simulink model "sim10"  (R2022b)
settings: Solver=VariableStepAuto  StartTime=0.0  StopTime=czas_symulacji  RelTol=1e-3
values from neighbouring files (symbols this model uses):
  Cvp = cp*rop*Vp    (= 36000)    [Lab5.m]    (also in Lab5_wspolne_wykresy.m)
  Cvw = cp*rop*Vw    (= 67200)    [Lab5.m]    (also in Lab5_wspolne_wykresy.m)
  dqg = 0.1*qgN    (= 1000)    [Lab5.m]    (also in Lab5_wspolne_wykresy.m)
  dTzew = 1    [Lab5.m]    (also in Lab5_wspolne_wykresy.m)
  kcp = (a*qgN*(TwewN-TpN))/((TpN-TzewN)*((TwewN-TzewN)+a*(TwewN-TpN)))    (= 23.2558139535)    [Lab5.m]    (also in Lab5_wspolne_wykresy.m)
  kcw = qgN/((TwewN-TzewN)+a*(TwewN-TpN))    (= 232.558139535)    [Lab5.m]    (also in Lab5_wspolne_wykresy.m)
  kcwp = a*kcw    (= 69.7674418605)    [Lab5.m]    (also in Lab5_wspolne_wykresy.m)
  L11 = M2    [Lab5.m]    (also in Lab5_wspolne_wykresy.m)
  L12 = [kcw*Cvp kcp*kcwp+kcw*kcwp+kcw*kcp]    [Lab5.m]    (also in Lab5_wspolne_wykresy.m)
  L21 = kcwp    (= 69.7674418605)    [Lab5.m]    (also in Lab5_wspolne_wykresy.m)
  L22 = [kcp*Cvw kcwp*kcw+kcw*kcp+kcwp*kcp]    [Lab5.m]    (also in Lab5_wspolne_wykresy.m)
  M = [Cvw*Cvp Cvw*kcwp+Cvw*kcp+Cvp*kcw+Cvp*kcwp kcw*kcwp+kcw*kcp+kcwp*kcp]    [Lab5.m]    (also in Lab5_wspolne_wykresy.m)
  qg0 = X(i)    [Lab5.m]    (also in Lab5_wspolne_wykresy.m)
  t0 = 1000    [Lab5.m]    (also in Lab5_wspolne_wykresy.m)
  Tp0 = ((kcp*Tzew0)*(kcw+kcwp)+kcwp*(qg0+kcw*Tzew0))/(kcwp*kcw+kcp*kcw+kcp*kcwp)    [Lab5.m]    (also in Lab5_wspolne_wykresy.m)
  Twew0 = (qg0+kcw*Tzew0+kcwp*Tp0)/(kcw+kcwp)    [Lab5.m]    (also in Lab5_wspolne_wykresy.m)
  Tzew0 = Y(i)    [Lab5.m]    (also in Lab5_wspolne_wykresy.m)
settings Model: Creator=franc  LastModifiedBy=Dawkin
settings DataIOCC: ReturnWorkspaceOutputs=off

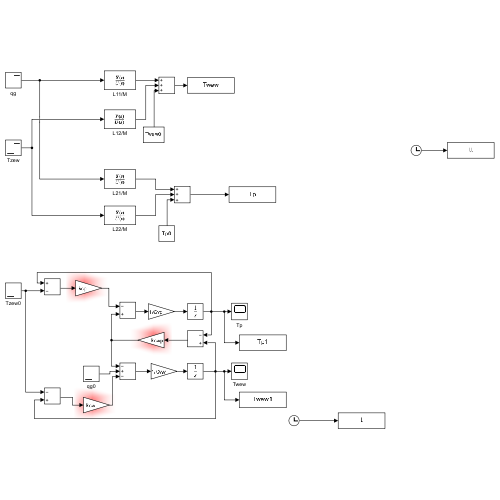
[thumbnail: Simulink's stored preview of the top-level diagram]
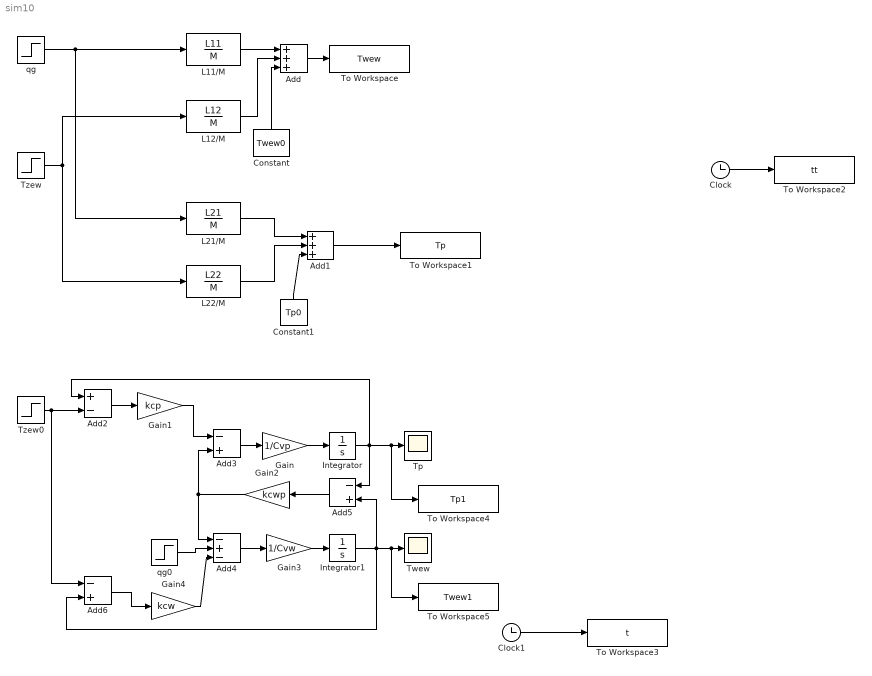
== system sim10 ==
  Add : Sum  Inputs=+++
  Add1 : Sum  Inputs=+++
  Add2 : Sum  Inputs=+-
  Add3 : Sum  Inputs=-+
  Add4 : Sum  Inputs=-+-
  Add5 : Sum  Inputs=-+
  Add6 : Sum  Inputs=-+
  Clock : Clock
  Clock1 : Clock
  Constant : Constant  Value=Twew0
  Constant1 : Constant  Value=Tp0
  Gain : Gain  Gain=1/Cvp
  Gain1 : Gain  Gain=kcp
  Gain2 : Gain  Gain=kcwp
  Gain3 : Gain  Gain=1/Cvw
  Gain4 : Gain  Gain=kcw
  Integrator : Integrator  InitialCondition=Tp0
  Integrator1 : Integrator  InitialCondition=Twew0
  L11/M : TransferFcn  Numerator=L11  Denominator=M
  L12/M : TransferFcn  Numerator=L12  Denominator=M
  L21/M : TransferFcn  Numerator=L21  Denominator=M
  L22/M : TransferFcn  Numerator=L22  Denominator=M
  To Workspace : ToWorkspace  VariableName=Twew  SampleTime=-1
  To Workspace1 : ToWorkspace  VariableName=Tp  SampleTime=-1
  To Workspace2 : ToWorkspace  VariableName=tt  SaveFormat=Timeseries  SampleTime=-1
  To Workspace3 : ToWorkspace  VariableName=t  SaveFormat=Timeseries  SampleTime=-1
  To Workspace4 : ToWorkspace  VariableName=Tp1  SampleTime=-1
  To Workspace5 : ToWorkspace  VariableName=Twew1  SampleTime=-1
  Tp : Scope
  Twew : Scope
  Tzew : Step  After=dTzew  SampleTime=0
  Tzew0 : Step  Time=t0  Before=Tzew0  After=Tzew0+dTzew  SampleTime=0
  qg : Step  After=dqg  SampleTime=0
  qg0 : Step  Time=t0  Before=qg0  After=qg0+dqg  SampleTime=0
  wires:
  qg/1 -> L21/M/1, L11/M/1
  L11/M/1 -> Add/1
  Tzew/1 -> L22/M/1, L12/M/1
  L12/M/1 -> Add/2
  Add/1 -> To Workspace/1
  L21/M/1 -> Add1/1
  L22/M/1 -> Add1/2
  Add1/1 -> To Workspace1/1
  Clock/1 -> To Workspace2/1
  Constant/1 -> Add/3
  Constant1/1 -> Add1/3
  Tzew0/1 -> Add2/2, Add6/1
  Add6/1 -> Gain4/1
  Gain4/1 -> Add4/3
  Clock1/1 -> To Workspace3/1
  Add4/1 -> Gain3/1
  qg0/1 -> Add4/2
  Integrator/1 -> To Workspace4/1, Tp/1, Add2/1, Add5/1
  Add5/1 -> Gain2/1
  Integrator1/1 -> Add6/2, Add5/2, To Workspace5/1, Twew/1
  Gain/1 -> Integrator/1
  Gain2/1 -> Add3/2, Add4/1
  Add3/1 -> Gain/1
  Gain3/1 -> Integrator1/1
  Add2/1 -> Gain1/1
  Gain1/1 -> Add3/1
